simulink model "CONTRO~1"  (R2019a)
settings: Solver=VariableStepAuto  StartTime=0.0  StopTime=10  RelTol=1e-3
values from neighbouring files (symbols this model uses):
  a = [0 1 0;0 0 1;-60 -11 -6]    [Controlador2_com_perturbacoes_planta_sem_integrador.m]
  A = [0 1 0;0 0 1;-6 -11 -6]    [Controlador2_com_perturbacoes_planta_sem_integrador.m]    (also in Q1_PCEEP3.m = [0 1 0; 0 0 1; 0 -200 -30]; Q2_PCEEP3.m = [0 1; -8 -4])
  B = [0 0 1]'    [Controlador2_com_perturbacoes_planta_sem_integrador.m]    (also in Q1_PCEEP3.m = [0; 0; 1]; Q2_PCEEP3.m = [0; 1])
  Kbar = acker(Abar,Bbar,polosMF)    [Controlador2_com_perturbacoes_planta_sem_integrador.m]
settings Model: Creator=rcard  LastModifiedBy=rcard

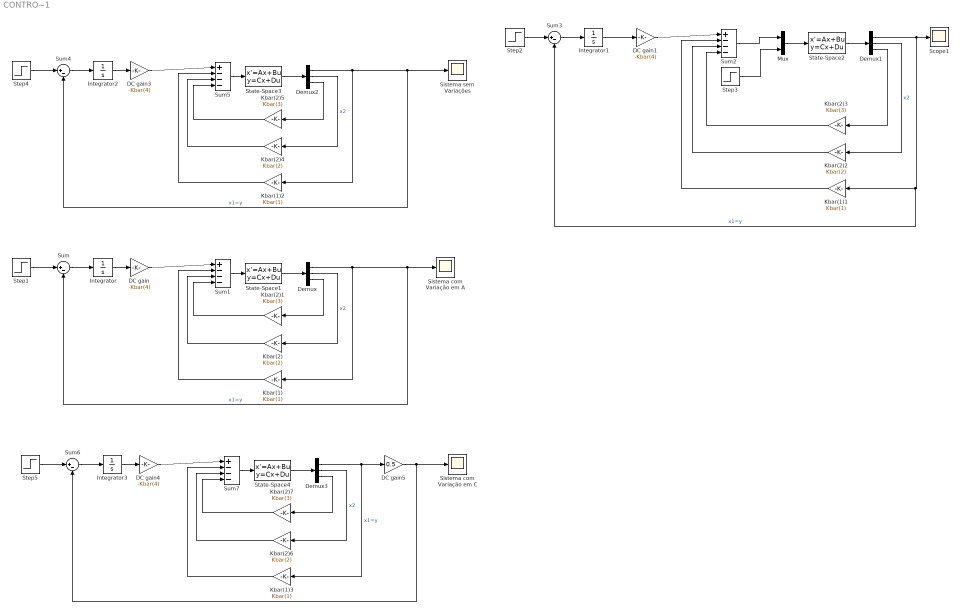
== system CONTRO~1 ==
  DC gain{,1,3..4} (4 alike) : Gain  Gain=-Kbar(4)
  DC gain5 : Gain  Gain=0.5
  Demux{,1..3} (4 alike) : Demux  Outputs=3
  Integrator{,1..3} (4 alike) : Integrator
  Kbar(1){,1..3} (4 alike) : Gain  Gain=Kbar(1)
  Kbar(2){,2,4,6} (4 alike) : Gain  Gain=Kbar(2)
  Kbar(2){1,3,5,7} (4 alike) : Gain  Gain=Kbar(3)
  Mux : Mux  Inputs=2
  Scope1 : Scope
  Sistema com Variação em A : Scope
  Sistema com Variação em C : Scope
  Sistema sem Variações : Scope
  State-Space1 : StateSpace  A=a  B=B  C=eye(3)  D=zeros(3,1)  InitialCondition=[0 0 0]
  State-Space2 : StateSpace  A=A  B=[B -B]  C=eye(3)  D=zeros(3,2)  InitialCondition=[0 0 0]
  State-Space3 : StateSpace  A=A  B=B  C=eye(3)  D=zeros(3,1)  InitialCondition=[0 0 0]
  State-Space4 : StateSpace  A=A  B=B  C=eye(3)  D=zeros(3,1)  InitialCondition=[0 0 0]
  Step{1..2,4..5} (4 alike) : Step  Time=0  SampleTime=1/20000
  Step3 : Step  Time=5  After=5  SampleTime=1/20000
  Sum{,3..4,6} (4 alike) : Sum  Inputs=|+-
  Sum{1..2,5,7} (4 alike) : Sum  Inputs=|+---
  wires:
  Sum1/1 -> State-Space1/1
  State-Space1/1 -> Demux/1
  Demux/1 -> Sum/2, Sistema com Variação em A/1, Kbar(1)/1  "x1=y"
  Demux/2 -> Kbar(2)/1  "x2"
  Kbar(2)/1 -> Sum1/3
  Kbar(1)/1 -> Sum1/2
  Demux/3 -> Kbar(2)1/1
  Kbar(2)1/1 -> Sum1/4
  DC gain/1 -> Sum1/1
  DC gain1/1 -> Sum2/1
  Kbar(2)2/1 -> Sum2/3
  State-Space2/1 -> Demux1/1
  Demux1/2 -> Kbar(2)2/1  "x2"
  Kbar(2)3/1 -> Sum2/4
  Demux1/3 -> Kbar(2)3/1
  Kbar(1)1/1 -> Sum2/2
  Demux1/1 -> Sum3/2, Kbar(1)1/1, Scope1/1  "x1=y"
  Mux/1 -> State-Space2/1
  Sum2/1 -> Mux/1
  Step3/1 -> Mux/2
  Step1/1 -> Sum/1
  Sum/1 -> Integrator/1
  Integrator/1 -> DC gain/1
  Step2/1 -> Sum3/1
  Sum3/1 -> Integrator1/1
  Integrator1/1 -> DC gain1/1
  Step4/1 -> Sum4/1
  Integrator2/1 -> DC gain3/1
  Sum5/1 -> State-Space3/1
  Sum4/1 -> Integrator2/1
  Kbar(2)5/1 -> Sum5/4
  Demux2/3 -> Kbar(2)5/1
  Demux2/2 -> Kbar(2)4/1  "x2"
  DC gain3/1 -> Sum5/1
  Kbar(1)2/1 -> Sum5/2
  Kbar(2)4/1 -> Sum5/3
  Demux2/1 -> Sum4/2, Sistema sem Variações/1, Kbar(1)2/1  "x1=y"
  State-Space3/1 -> Demux2/1
  Step5/1 -> Sum6/1
  Integrator3/1 -> DC gain4/1
  Sum7/1 -> State-Space4/1
  DC gain5/1 -> Sum6/2, Sistema com Variação em C/1
  Sum6/1 -> Integrator3/1
  Kbar(2)7/1 -> Sum7/4
  Demux3/3 -> Kbar(2)7/1
  Demux3/2 -> Kbar(2)6/1  "x2"
  DC gain4/1 -> Sum7/1
  Kbar(1)3/1 -> Sum7/2
  Kbar(2)6/1 -> Sum7/3
  Demux3/1 -> Kbar(1)3/1, DC gain5/1  "x1=y"
  State-Space4/1 -> Demux3/1
